simulink model "epidemia"  (R2020b)
settings: Solver=VariableStepAuto  StartTime=0.0  StopTime=200  RelTol=1e-3
settings Model: Creator=matis  LastModifiedBy=matis

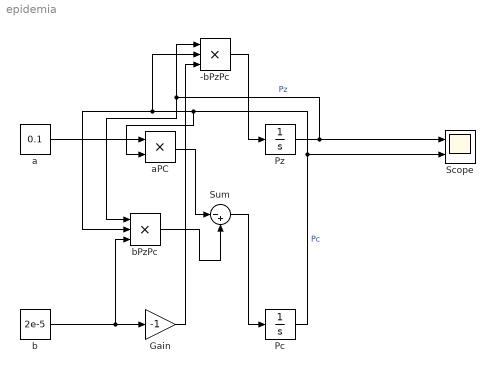
== system epidemia ==
  -bPzPc : Product  Inputs=3
  Gain : Gain  Gain=-1
  Pc : Integrator  InitialCondition=10
  Pz : Integrator  InitialCondition=10000
  Scope : Scope  NumInputPorts=2
  Sum : Sum  Inputs=|-+
  a : Constant  Value=0.1
  aPC : Product
  b : Constant  Value=2e-5
  bPzPc : Product  Inputs=3
  wires:
  Pz/1 -> Scope/1, bPzPc/1, -bPzPc/1  "Pz"
  Pc/1 -> Scope/2, aPC/2, bPzPc/2, -bPzPc/2  "Pc"
  b/1 -> bPzPc/3, Gain/1
  Gain/1 -> -bPzPc/3
  -bPzPc/1 -> Pz/1
  a/1 -> aPC/1
  bPzPc/1 -> Sum/2
  aPC/1 -> Sum/1
  Sum/1 -> Pc/1
